simulink subsystem "NoBMS"  (R2023b)
settings: Solver=VariableStepAuto  StartTime=0.0  StopTime=10.0  RelTol=1e-3
settings Model: Creator=The MathWorks, Inc.  LastModifiedBy=The MathWorks, Inc.

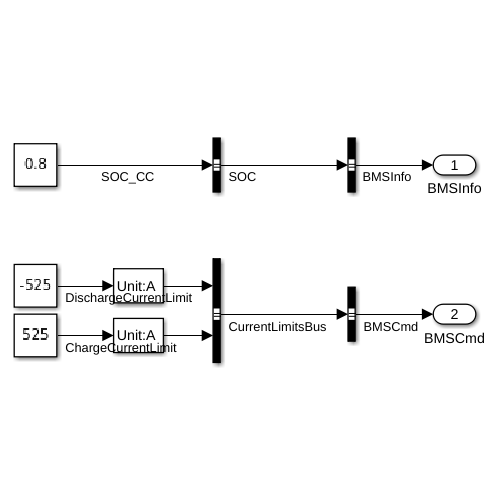
[thumbnail: Simulink's stored preview of the top-level diagram]
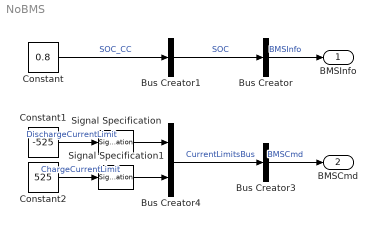
== system NoBMS ==
  Bus Creator : BusCreator  Inputs=1
  Bus Creator1 : BusCreator  Inputs=1
  Bus Creator3 : BusCreator  Inputs=1
  Bus Creator4 : BusCreator  Inputs=2
  Constant : Constant  Value=0.8  SampleTime=-1
  Constant1 : Constant  Value=-525  SampleTime=-1
  Constant2 : Constant  Value=525  SampleTime=-1
  Signal Specification : SignalSpecification  Unit=A
  Signal Specification1 : SignalSpecification  Unit=A
  BMSInfo : Outport
  BMSCmd : Outport  Port=2
  wires:
  Bus Creator/1 -> BMSInfo/1  "BMSInfo"
  Bus Creator1/1 -> Bus Creator/1  "SOC"
  Constant/1 -> Bus Creator1/1  "SOC_CC"
  Bus Creator3/1 -> BMSCmd/1  "BMSCmd"
  Bus Creator4/1 -> Bus Creator3/1  "CurrentLimitsBus"
  Constant1/1 -> Signal Specification/1  "DischargeCurrentLimit"
  Constant2/1 -> Signal Specification1/1  "ChargeCurrentLimit"
  Signal Specification/1 -> Bus Creator4/1
  Signal Specification1/1 -> Bus Creator4/2
